simulink model "photovoltaic"  (R2016b)
settings: Solver=ode45  StartTime=0.0  StopTime=40.0  RelTol=1e-3  EnableMultiTasking=on
libraries: fl_lib x6, nesl_utility x4, simulink x3, elec_lib x1, pe_lib x1
settings Model: Creator=Aluno IC  LastModifiedBy=icaro
settings DataIOCC: LimitDataPoints=on  SaveFormat=Array
settings OptimizationCC: LifeSpan=inf
settings DebuggingCC: SFUnexpectedBacktrackingDiag=warning  SFNoUnconditionalDefaultTransitionDiag=warning  SFExecutionAtInitializationDiag=none
settings HardwareCC: ProdBitPerPointer=32  ProdBitPerSizeT=32  ProdBitPerPtrDiffT=32  ProdLargestAtomicFloat=None  ProdIntDivRoundTo=Undefined  ProdEndianess=Unspecified  ProdWordSize=32  ProdHWDeviceType=32-bit Generic
settings ModelReferenceCC: PropagateSignalLabelsOutOfModel=off
settings GRTTargetCC: TargetLangStandard=C89/C90 (ANSI)  GeneratePreprocessorConditionals=Disable all
settings ConfigComp: CovMetricSettings=dw  CovHtmlReporting=on  CovSaveCumulativeToWorkspaceVar=on  CovSaveSingleToWorkspaceVar=on  CovExternalEMLEnable=off

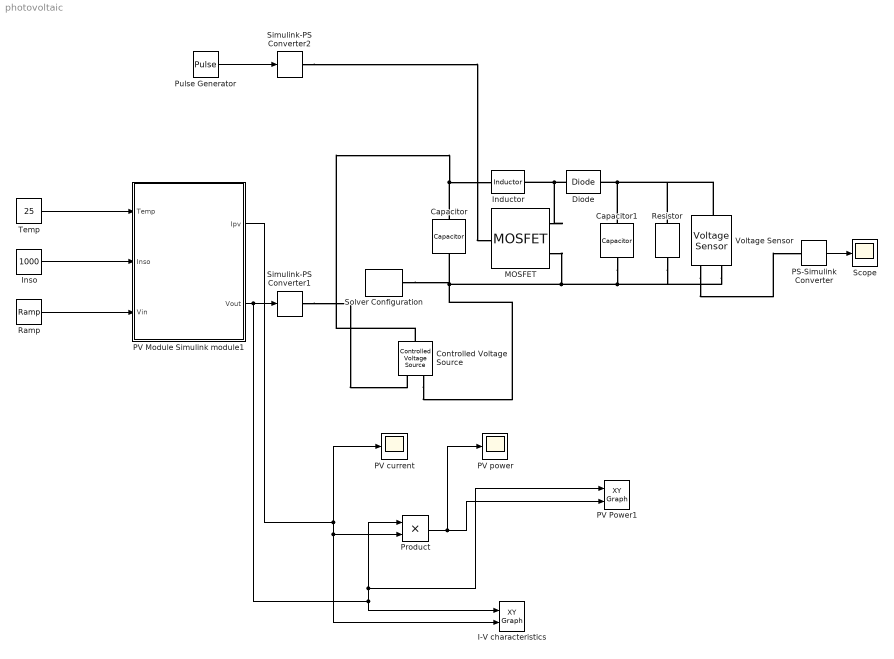
== system photovoltaic ==
  Capacitor : fl_lib/Electrical/Electrical Elements/Capacitor  c=1e-6 F  r=1e-6 Ohm  g=0 1/Ohm  i_specify=off  i_priority=None  i=0 A  v_specify=off  v_priority=None  v=0 V  vc_specify=off  vc_priority=High  vc=0 V
  Capacitor1 : fl_lib/Electrical/Electrical Elements/Capacitor  c=1e-6 F  r=1e-6 Ohm  g=0 1/Ohm  i_specify=off  i_priority=None  i=0 A  v_specify=off  v_priority=None  v=0 V  vc_specify=off  vc_priority=High  vc=0 V
  Controlled Voltage Source : fl_lib/Electrical/Electrical Sources/Controlled Voltage Source
  Diode : elec_lib/Semiconductor Devices/Diode  ModelType=1  Vf=0.6 V  Ron=0.3 Ohm  Goff=1e-8 S  Rz=0.3 Ohm  Vz=50 V  C_PWL=5 pF  prmExp=1  I12=[ 0.0137 0.545 ] A  V12=[ 0.6 0.7 ] V  I1=0.0137 A  V1=0.6 V  RS=0.01 Ohm  IS=1e-12 A  Tmeas=25 degC  ec=1  BV=Inf V  C_param=1  CJ0=5 pF  VJ=1 V  Mgrad=0.5  Vvec=[ 0.1 10 100 ] V  Cvec=[ 3.5 1 0.4 ] pF  FC=0.5  Q_param=1  Irrm=-7.15 A  iF=4 A  didt=-750 A/us  trr=115 ns  TT=50 ns  tau=100 ns  T_param=1  IS_T2=1.25e-7 A  I1_T2=0.245 A  V1_T2=0.5 V  Tmeas2=125 degC  EG_param=1  EG=1.11 eV  XTI_param=1  XTI=3  dBVdT=0 V/K  Tdevice=25 degC  Rth=[ 0 10 ] K/W  thermal_mass_parameterization=1  thermal_mass=[ 0 1 ] J/K  thermal_time_constant=[ 0 10 ] s  thermal_mass_initial_temperatures=[ 25 25 ] degC
  I-V characteristics : simulink/Sinks/XY Graph  xmin=-1  xmax=40  ymin=-1  ymax=40  st=-1
  Inductor : fl_lib/Electrical/Electrical Elements/Inductor  l=1e-6 H  r=0 Ohm  g=1e-9 1/Ohm  i_specify=off  i_priority=None  i=0 A  v_specify=off  v_priority=None  v=0 V  i_L_specify=off  i_L_priority=High  i_L=0 A
  Inso : Constant  Value=1000
  MOSFET : pe_lib/Semiconductors/Fundamental Components/MOSFET  Rds=0.01 Ohm  Goff=1e-6 1/Ohm  Vth=2 V  diode_param=2  diode_Vf=0.8 V  diode_Ron=0.001 Ohm  diode_Goff=1e-5 1/Ohm  diode_C=5e-8 F  diode_iRM=-235 A  diode_iF=300 A  diode_idot=-50 A/us  diode_trr_param=1  diode_trr_factor=3  diode_trr=15 us  diode_Qrr=1.5e+3 s*uA  thermal_loss_option=2  Voff=300 V  Tau=1e-4 s  Tj=[ 298.15 398.15 ] K  Iout_scalar=600 A  Eon_scalar=0.02286 J  Eoff_scalar=0.01714 J  Von_scalar=2.7 V  Iout_data=[ 0 10 50 100 200 400 600 ] A  Eon_data=[ 0 2.9e-4 0.00143 0.00286 0.00571 0.01314 0.02286; 0 5.7e-4 0.00263 0.00514 0.01029 0.02057 0.03029 ] J  Eoff_data=[ 0 2.1e-4 0.00107 0.00214 0.00429 0.009859999999999999 0.01714; 0 4.3e-4 0.00197 0.00386 0.00771 0.01543 0.02271 ] J  Von_data=[ 0 1.1 1.3 1.45 1.75 2.25 2.7; 0 1 1.15 1.35 1.7 2.35 3 ] V
  PS-Simulink Converter : nesl_utility/PS-Simulink Converter  PhysicalDomain=network_engine_domain  SubClassName=ps_output  LeftPortType=input  RightPortType=output  PseudoPeriodic=off  Frequencies=[]  Unit=1  AffineConversion=off
  PV Module Simulink module1 : Subsystem
  PV Power1 : simulink/Sinks/XY Graph  xmin=-1  xmax=40  ymin=-1  ymax=40  st=-1
  PV current : Scope
  "PV power " : Scope
  Product : Product
  Pulse Generator : DiscretePulseGenerator  PulseType=Time based  Period=1/25000  PulseWidth=60
  Ramp : simulink/Sources/Ramp  slope=1  start=0  X0=0
  Resistor : fl_lib/Electrical/Electrical Elements/Resistor  R=1 Ohm  i_specify=off  i_priority=None  i=0 A  v_specify=off  v_priority=None  v=0 V
  Scope : Scope
  Simulink-PS Converter1 : nesl_utility/Simulink-PS Converter  PhysicalDomain=network_engine_domain  SubClassName=ps_input  LeftPortType=input  RightPortType=output  PseudoPeriodic=off  Frequencies=[]  NoiseDistribution=none  NoiseParameters=[]  Unit=1  AffineConversion=off  InputFiltering=off  SimscapeFilterOrder=1  InputFilterTimeConstant=0.001  UdotUserProvided=1
  Simulink-PS Converter2 : nesl_utility/Simulink-PS Converter  PhysicalDomain=network_engine_domain  SubClassName=ps_input  LeftPortType=input  RightPortType=output  PseudoPeriodic=off  Frequencies=[]  NoiseDistribution=none  NoiseParameters=[]  Unit=1  AffineConversion=off  InputFiltering=off  SimscapeFilterOrder=1  InputFilterTimeConstant=0.001  UdotUserProvided=1
  Solver Configuration : nesl_utility/Solver Configuration  PhysicalDomain=network_engine_domain  SubClassName=solver  LeftPortType=input  RightPortType=generic  Accelerate=off  Tones=[]  Harmonics=[]  SimulateNoise=off  Profile=off  UseLocalSampling=off  EnableSwitchedLinearOptims=on  FrequencyDomain=off  UseCCode=off  RelTol=0.001  AbsTol=1e-06  MinStep=1e-09  ToWorkspace=off  RevertToSquareIcSolve=off  NumHomotopyIterations=100  PhasorMode=off  PhasorModeNumHarmonics=1  OverrideAbsTol=off  DoDC=off  ResidualTolerance=1e-09  UseLocalSolver=off  LocalSolverChoice=NE_BACKWARD_EULER_ADVANCER  LocalSolverSampleTime=0.001  DoFixedCost=off  MaxNonlinIter=3  MaxModeIter=2  LinearAlgebra=Sparse  DelaysMemoryBudget=1024  AutomaticFiltering=on  FilteringTimeConstant=0.001
  Temp : Constant  Value=25
  Voltage Sensor : fl_lib/Electrical/Electrical Sensors/Voltage Sensor
  wires:
  Inso/1 -> PV Module Simulink module1/2(Inso)
  Temp/1 -> PV Module Simulink module1/1(Temp)
  Pulse Generator/1 -> Simulink-PS Converter2/1
  PS-Simulink Converter/1 -> Scope/1
  Ramp/1 -> PV Module Simulink module1/3(Vin)
  PV Module Simulink module1/1(Ipv) -> I-V characteristics/2, Product/2, PV current/1
  Product/1 -> "PV power "/1, PV Power1/2
  PV Module Simulink module1/2(Vout) -> PV Power1/1, Product/1, I-V characteristics/1, Simulink-PS Converter1/1
  connections:
  Capacitor/LConn1 -- Controlled Voltage Source/LConn1 -- Inductor/LConn1
  Diode/LConn1 -- MOSFET/RConn1 -- Inductor/RConn1
  MOSFET/RConn2 -- Voltage Sensor/RConn2 -- Resistor/RConn1 -- Capacitor1/RConn1 -- Solver Configuration/RConn1 -- Capacitor/RConn1 -- Controlled Voltage Source/RConn2
  Simulink-PS Converter1/RConn1 -- Controlled Voltage Source/RConn1
  Simulink-PS Converter2/RConn1 -- MOSFET/LConn1
  Capacitor1/LConn1 -- Voltage Sensor/LConn1 -- Resistor/LConn1 -- Diode/RConn1
  Voltage Sensor/RConn1 -- PS-Simulink Converter/LConn1

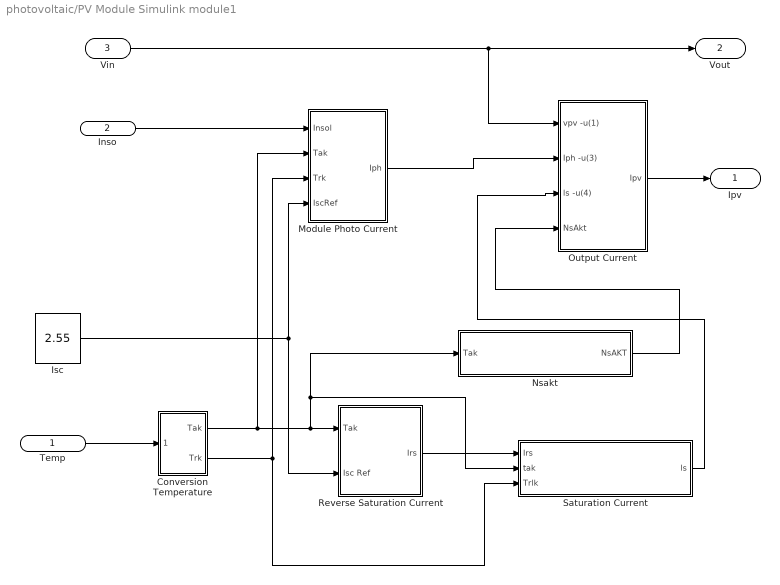
== system photovoltaic/PV Module Simulink module1 ==
  Temp : Inport
  Inso : Inport  Port=2
  Vin : Inport  Port=3
  Conversion Temperature : Subsystem
  Isc : Constant  Value=2.55
  Module Photo Current : Subsystem
  "Nsakt " : Subsystem
  "Output Current " : Subsystem
  Reverse Saturation Current : Subsystem
  Saturation Current : Subsystem
  Ipv : Outport
  Vout : Outport  Port=2
  wires:
  Conversion Temperature/1("Tak ") -> Module Photo Current/2("Tak "), "Nsakt "/1(Tak), Saturation Current/2(tak), Reverse Saturation Current/1(Tak)
  Saturation Current/1(ls) -> "Output Current "/3(ls -u(4))
  "Nsakt "/1("NsAKT ") -> "Output Current "/4(NsAkt)
  Module Photo Current/1(Iph) -> "Output Current "/2(Iph -u(3))
  Conversion Temperature/2(Trk) -> Saturation Current/3(Trlk), Module Photo Current/3("Trk ")
  Temp/1 -> Conversion Temperature/1("Top ")
  Inso/1 -> Module Photo Current/1(Insol)
  Reverse Saturation Current/1(Irs) -> Saturation Current/1("Irs ")
  Vin/1 -> Vout/1, "Output Current "/1(vpv -u(1))
  Isc/1 -> Module Photo Current/4(IscRef), Reverse Saturation Current/2(Isc Ref)
  "Output Current "/1(Ipv) -> Ipv/1

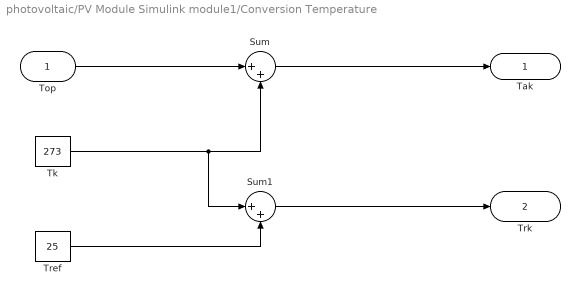
== system photovoltaic/PV Module Simulink module1/Conversion Temperature ==
  "Top " : Inport
  Sum : Sum  Inputs=|++
  Sum1 : Sum  Inputs=|++
  Tk : Constant  Value=273
  Tref : Constant  Value=25
  "Tak " : Outport
  Trk : Outport  Port=2
  wires:
  Sum1/1 -> Trk/1
  Tref/1 -> Sum1/2
  "Top "/1 -> Sum/1
  Tk/1 -> Sum1/1, Sum/2
  Sum/1 -> "Tak "/1

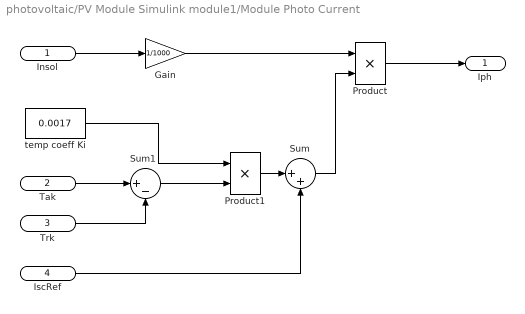
== system photovoltaic/PV Module Simulink module1/Module Photo Current ==
  Insol : Inport
  "Tak " : Inport  Port=2
  "Trk " : Inport  Port=3
  IscRef : Inport  Port=4
  Gain : Gain  Gain=1/1000
  Product : Product
  Product1 : Product
  Sum : Sum  Inputs=|++
  Sum1 : Sum  Inputs=|+-
  temp coeff Ki : Constant  Value=0.0017
  Iph : Outport
  wires:
  IscRef/1 -> Sum/2
  Gain/1 -> Product/1
  Sum1/1 -> Product1/2
  Product1/1 -> Sum/1
  Product/1 -> Iph/1
  "Tak "/1 -> Sum1/1
  Sum/1 -> Product/2
  "Trk "/1 -> Sum1/2
  temp coeff Ki/1 -> Product1/1
  Insol/1 -> Gain/1

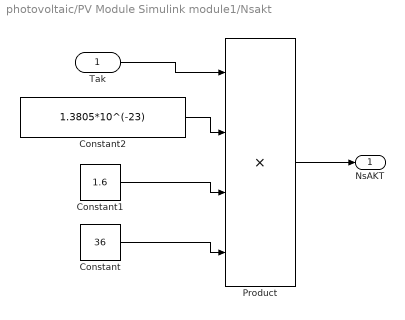
== system photovoltaic/PV Module Simulink module1/Nsakt  ==
  Tak : Inport
  Constant : Constant  Value=36
  Constant1 : Constant  Value=1.6
  Constant2 : Constant  Value=1.3805*10^(-23)
  Product : Product  Inputs=4
  "NsAKT " : Outport
  wires:
  Product/1 -> "NsAKT "/1
  Constant2/1 -> Product/2
  Constant1/1 -> Product/3
  Constant/1 -> Product/4
  Tak/1 -> Product/1

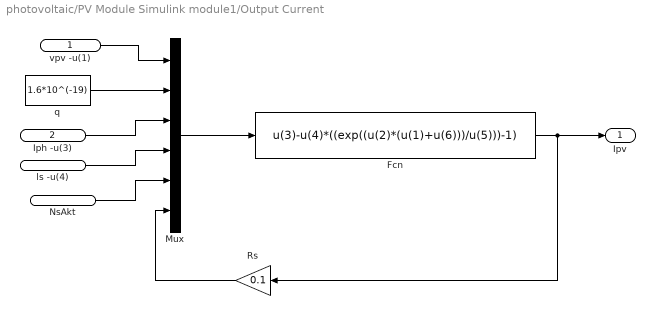
== system photovoltaic/PV Module Simulink module1/Output Current  ==
  vpv -u(1) : Inport
  Iph -u(3) : Inport  Port=2
  ls -u(4) : Inport  Port=3
  NsAkt : Inport  Port=4
  Fcn : Fcn  Expr=u(3)-u(4)*((exp((u(2)*(u(1)+u(6)))/u(5)))-1)
  Mux : Mux  Inputs=6
  Rs : Gain  Gain=0.1
  q : Constant  Value=1.6*10^(-19)
  Ipv : Outport
  wires:
  q/1 -> Mux/2
  Rs/1 -> Mux/6
  Iph -u(3)/1 -> Mux/3
  ls -u(4)/1 -> Mux/4
  NsAkt/1 -> Mux/5
  vpv -u(1)/1 -> Mux/1
  Fcn/1 -> Ipv/1, Rs/1
  Mux/1 -> Fcn/1

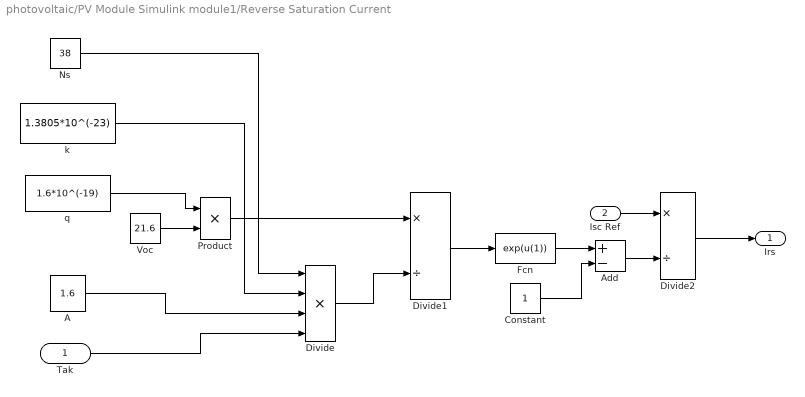
== system photovoltaic/PV Module Simulink module1/Reverse Saturation Current ==
  Tak : Inport
  Isc Ref : Inport  Port=2
  A : Constant  Value=1.6
  Add : Sum  Inputs=+-
  Constant : Constant
  Divide : Product  Inputs=4
  Divide1 : Product  Inputs=*/
  Divide2 : Product  Inputs=*/
  Fcn : Fcn  Expr=exp(u(1))
  Ns : Constant  Value=38
  Product : Product
  Voc : Constant  Value=21.6
  k : Constant  Value=1.3805*10^(-23)
  q : Constant  Value=1.6*10^(-19)
  Irs : Outport
  wires:
  Divide2/1 -> Irs/1
  Ns/1 -> Divide/1
  Isc Ref/1 -> Divide2/1
  Divide1/1 -> Fcn/1
  Product/1 -> Divide1/1
  k/1 -> Divide/2
  A/1 -> Divide/3
  Divide/1 -> Divide1/2
  Tak/1 -> Divide/4
  Add/1 -> Divide2/2
  Fcn/1 -> Add/1
  Constant/1 -> Add/2
  q/1 -> Product/1
  Voc/1 -> Product/2

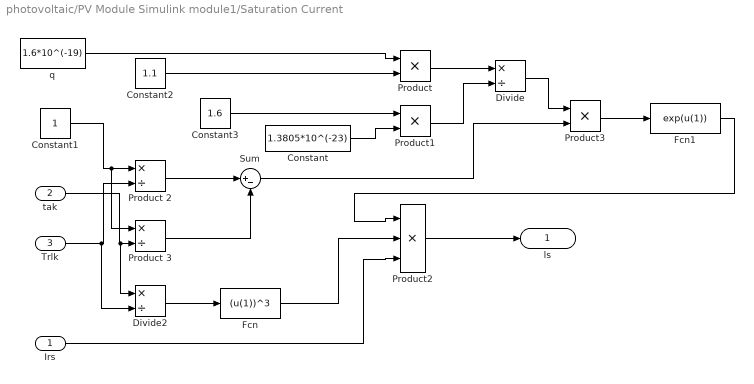
== system photovoltaic/PV Module Simulink module1/Saturation Current ==
  "Irs " : Inport
  tak : Inport  Port=2
  Trlk : Inport  Port=3
  Constant : Constant  Value=1.3805*10^(-23)
  Constant1 : Constant
  Constant2 : Constant  Value=1.1
  Constant3 : Constant  Value=1.6
  Divide : Product  Inputs=*/
  Divide2 : Product  Inputs=*/
  Fcn : Fcn  Expr=(u(1))^3
  Fcn1 : Fcn  Expr=exp(u(1))
  Product : Product
  Product 2 : Product  Inputs=*/
  Product 3 : Product  Inputs=*/
  Product1 : Product
  Product2 : Product  Inputs=3
  Product3 : Product
  Sum : Sum  Inputs=|+-
  q : Constant  Value=1.6*10^(-19)
  ls : Outport
  wires:
  Constant2/1 -> Product/2
  Product3/1 -> Fcn1/1
  "Irs "/1 -> Product2/3
  q/1 -> Product/1
  Fcn/1 -> Product2/2
  Divide2/1 -> Fcn/1
  Product 2/1 -> Sum/1
  Product 3/1 -> Sum/2
  Product2/1 -> ls/1
  Product/1 -> Divide/1
  Constant3/1 -> Product1/1
  Sum/1 -> Product3/2
  Product1/1 -> Divide/2
  Constant/1 -> Product1/2
  Fcn1/1 -> Product2/1
  Divide/1 -> Product3/1
  Trlk/1 -> Product 2/2, Divide2/2
  tak/1 -> Divide2/1, Product 3/2
  Constant1/1 -> Product 3/1, Product 2/1
